simulink model "ex4_dcmotor_with_controller"  (R2025b)
settings: Solver=VariableStepAuto  StartTime=0.0  StopTime=0.01  RelTol=1e-3
values from neighbouring files (symbols this model uses):
  par = param_setter(0.23*10^(-3), 23.4*10^(-3), 2.4, 0.23*10^(-6), 0.4191*10^(-5))    [model_runner.m]
libraries: cstblocks x2
settings Model: Creator=fred  LastModifiedBy=fred

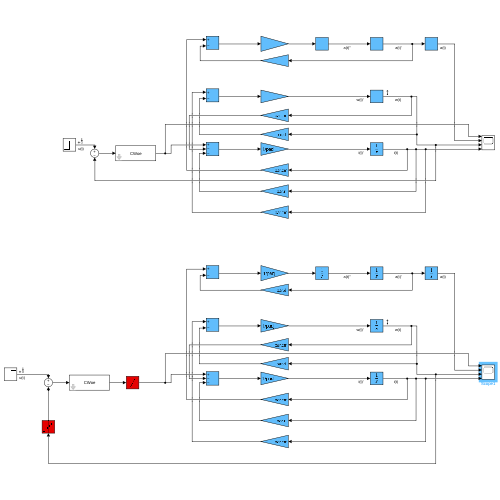
[thumbnail: Simulink's stored preview of the top-level diagram]
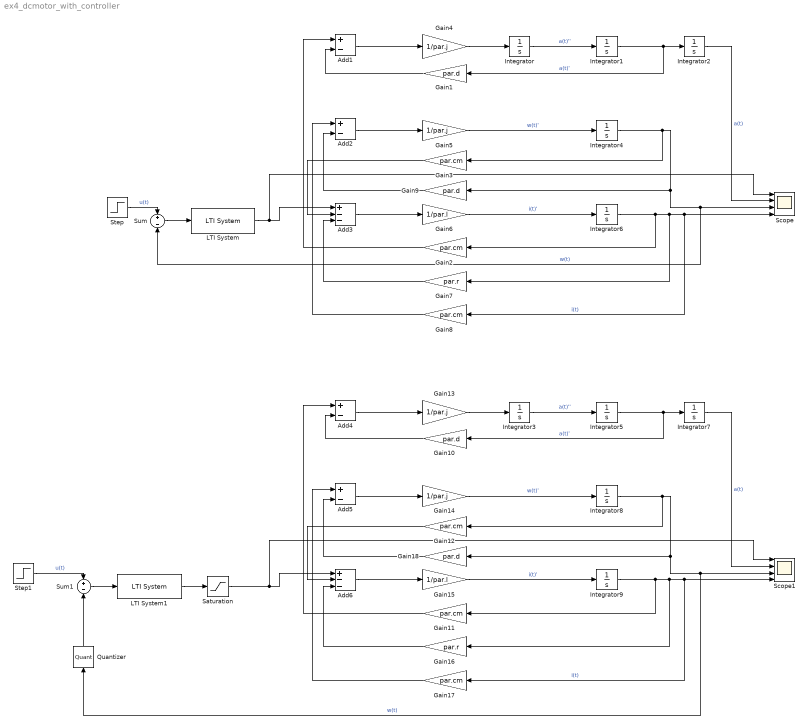
== system ex4_dcmotor_with_controller ==
  Add{1..2,4..5} (4 alike) : Sum  Inputs=+-
  Add3 : Sum  Inputs=+--
  Add6 : Sum  Inputs=+--
  Gain{1,9..10,18} (4 alike) : Gain  Gain=par.d
  Gain{2..3,8,11..12,17} (6 alike) : Gain  Gain=par.cm
  Gain{4..5,13..14} (4 alike) : Gain  Gain=1/par.j
  Gain15 : Gain  Gain=1/par.l
  Gain16 : Gain  Gain=par.r
  Gain6 : Gain  Gain=1/par.l
  Gain7 : Gain  Gain=par.r
  Integrator{,1..9} (10 alike) : Integrator
  LTI System : cstblocks/LTI System  sys=CWoe  IC=[]  PadeOrder=0
  LTI System1 : cstblocks/LTI System  sys=CWoe  IC=[]  PadeOrder=0
  Quantizer : Quantizer
  Saturation : Saturate  UpperLimit=12  LowerLimit=-12
  Scope : Scope  NumInputPorts=4
      settings: ActiveDisplayYMinimum=-10.083907468634075  ActiveDisplayYMaximum=13.207966054025873  DataLoggingVariableName=output
  Scope1 : Scope  NumInputPorts=4
      settings: ActiveDisplayYMinimum=-4.4845808055251837  ActiveDisplayYMaximum=14.268709183573737  DataLoggingVariableName=output1
  Step : Step  Time=0  After=314  SampleTime=0
  Step1 : Step  Time=0  After=314  SampleTime=0
  Sum : Sum  Inputs=+-
  Sum1 : Sum  Inputs=+-
  wires:
  Integrator1/1 -> Gain1/1, Integrator2/1  "a(t)'"
  Integrator/1 -> Integrator1/1  "a(t)''"
  Integrator2/1 -> Scope/2  "a(t)"
  Integrator4/1 -> Scope/3, Sum/2, Gain9/1, Gain3/1  "w(t)"
  Gain6/1 -> Integrator6/1  "i(t)'"
  Integrator6/1 -> Gain2/1, Gain8/1, Scope/4, Gain7/1  "i(t)"
  Gain1/1 -> Add1/2
  Gain2/1 -> Add1/1
  Add1/1 -> Gain4/1
  Gain4/1 -> Integrator/1
  Add2/1 -> Gain5/1
  Add3/1 -> Gain6/1
  Gain7/1 -> Add3/3
  Gain3/1 -> Add3/2
  Gain8/1 -> Add2/1
  Gain9/1 -> Add2/2
  Gain5/1 -> Integrator4/1  "w(t)'"
  Step/1 -> Sum/1  "u(t)"
  Sum/1 -> LTI System/1
  LTI System/1 -> Scope/1, Add3/1
  Add6/1 -> Gain15/1
  Add5/1 -> Gain14/1
  Gain11/1 -> Add4/1
  Gain10/1 -> Add4/2
  Integrator9/1 -> Gain11/1, Gain17/1, Scope1/4, Gain16/1  "i(t)"
  Gain15/1 -> Integrator9/1  "i(t)'"
  Integrator8/1 -> Scope1/3, Quantizer/1, Gain18/1, Gain12/1  "w(t)"
  Sum1/1 -> LTI System1/1
  Integrator3/1 -> Integrator5/1  "a(t)''"
  Step1/1 -> Sum1/1  "u(t)"
  LTI System1/1 -> Saturation/1
  Gain17/1 -> Add5/1
  Gain18/1 -> Add5/2
  Gain14/1 -> Integrator8/1  "w(t)'"
  Gain13/1 -> Integrator3/1
  Integrator5/1 -> Gain10/1, Integrator7/1  "a(t)'"
  Gain12/1 -> Add6/2
  Integrator7/1 -> Scope1/2  "a(t)"
  Gain16/1 -> Add6/3
  Add4/1 -> Gain13/1
  Saturation/1 -> Scope1/1, Add6/1
  Quantizer/1 -> Sum1/2
